simulink model "Orbit_prop_279C_v2"  (R2018b)
settings: Solver=FixedStepAuto  StartTime=0.0  StopTime=3600*24*177*omega  FixedStep=25*omega  MaxStep=25*omega  RelTol=1e-10  AbsTol=1e-12
values from neighbouring files (symbols this model uses):
  mu1 = 328900.56^-1    (= 3.04043264627e-06)    [Compare_run.m]    (also in PSet1.m; Pset3_Orbit_prop.m; Pset3_Orbit_prop_dim.m; Pset_4_TD.m)
  r0 = [.98900883730044109; 0; 0.000802140914099732]*dis.sun    [Compare_run.m]    (also in Pset3_Orbit_prop.m = [.98900883730044109; 0; 0.000802140914099732]; Pset3_Orbit_prop_dim.m; Pset_4_TD.m; Sim_Run_File.m)
  v0 = [0; 0.010697471710460349-2.895683e-3; 0] * dis.sun * omega    [Compare_run.m]    (also in Pset3_Orbit_prop.m = [0; 0.010697471710460349-3.24371e-3; 0]; Pset3_Orbit_prop_dim.m; Pset_4_TD.m; Sim_Run_File.m)
settings Model: Creator=ayotundedemuren  LastModifiedBy=Ethan
settings SolverCC: AutoScaleAbsTol=off

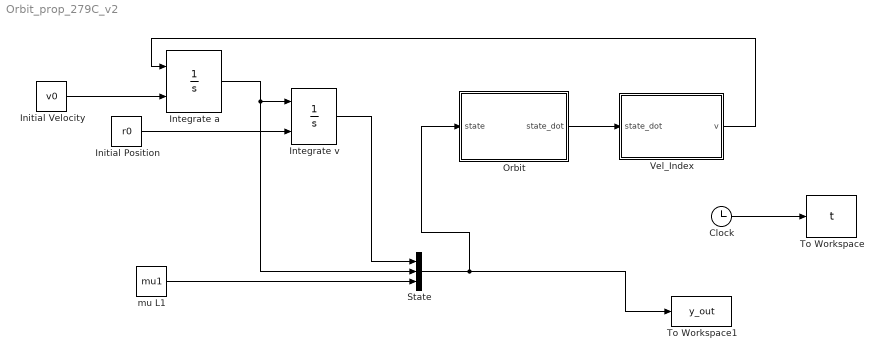
== system Orbit_prop_279C_v2 ==
  Clock : Clock
  Initial Position : Constant  Value=r0
  Initial Velocity : Constant  Value=v0
  Integrate a : Integrator  InitialConditionSource=external  AbsoluteTolerance=1e-6
  Integrate v : Integrator  InitialConditionSource=external  AbsoluteTolerance=1e-6
  Orbit : MATLAB Function  TreatAsAtomicUnit=on
  "State " : Concatenate  NumInputs=3
  To Workspace : ToWorkspace  VariableName=t  SampleTime=-1
      settings: Save2DSignal=2-D array (concatenate along first dimension)
  To Workspace1 : ToWorkspace  VariableName=y_out  SampleTime=-1
  Vel_Index : MATLAB Function  TreatAsAtomicUnit=on
  mu L1 : Constant  Value=mu1
  wires:
  Initial Velocity/1 -> Integrate a/2
  Initial Position/1 -> Integrate v/2
  Integrate v/1 -> "State "/1
  Vel_Index/1(v) -> Integrate a/1
  "State "/1 -> Orbit/1(state), To Workspace1/1
  Integrate a/1 -> Integrate v/1, "State "/2
  mu L1/1 -> "State "/3
  Orbit/1(state_dot) -> Vel_Index/1(state_dot)
  Clock/1 -> To Workspace/1

== matlab function Orbit_prop_279C_v2/Vel_Index ==
  data: state_dot input; v output
function v = fcn(state_dot)

v = state_dot(4:6);

end

== matlab function Orbit_prop_279C_v2/Orbit ==
  data: state input; state_dot output
function state_dot = fcn(state)

state_dot = zeros(7,1);
x = state(1);
y = state(2);
z = state(3);
xdot = state(4);
ydot = state(5);
zdot = state(6);

mu = state(7);

rho1 = sqrt((x + mu)^2 + y^2 + z^2);
rho2 = sqrt((x - (1-mu))^2 + y^2 + z^2);

state_dot(1) = xdot;
state_dot(2) = ydot;
state_dot(3) = zdot;

state_dot(4) = x + 2*ydot - (1 - mu)*(x + mu)/rho1^3 - ...
    mu*(x - (1 - mu))/rho2^3;
state_dot(5) = y - 2*xdot - (1 - mu)*(y)/rho1^3 - ...
    mu*(y)/rho2^3;
state_dot(6) = -(1 - mu)*z/rho1^3 - mu*z/rho2^3;
for ii = 4:6
    if abs(state_dot(ii)) < 1e-15
        state_dot(ii) = 0;
    end
end
end
